simulink model "transmitSim"  (R2019a)
settings: Solver=VariableStepAuto  StartTime=0.0  StopTime=0.01  RelTol=1e-3
values from neighbouring files (symbols this model uses):
  data = 1:53    [cable.m]
libraries: commrandsrc3 x2, commdigbbndam3 x2, rfports1 x2, commchan3 x1, rftxlines1 x1
settings Model: Creator=PABLO  LastModifiedBy=PABLO

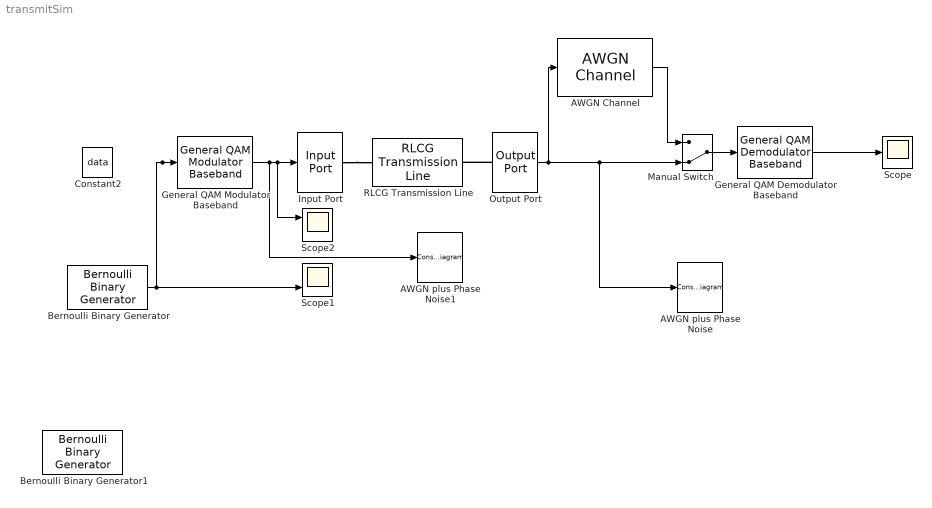
== system transmitSim ==
  AWGN Channel : commchan3/AWGN Channel  InputProcessing=Columns as channels (frame based)  seed=67  noiseMode="Signal to noise ratio  (Eb/No)"  EbNodB=10  EsNodB=10  SNRdB=10  bitsPerSym=1  Ps=1  Tsym=1  variance=1
      settings: SourceProductName=Communications Toolbox
  AWGN plus Phase Noise : ConstellationDiagram  Tag=ScatterPlot
  AWGN plus Phase Noise1 : ConstellationDiagram  Tag=ScatterPlot
  Bernoulli Binary Generator : commrandsrc3/Bernoulli Binary Generator  ProbabilityOfZero=0.5  SeedSource=Auto  Seed=0  SampleTime=1e-7  SamplesPerFrame=1  OutputDataType=double  SimulateUsing=Interpreted execution
      settings: SourceProductName=Communications Toolbox
  Bernoulli Binary Generator1 : commrandsrc3/Bernoulli Binary Generator  ProbabilityOfZero=0.5  SeedSource=Auto  Seed=0  SampleTime=1e-7  SamplesPerFrame=1  OutputDataType=boolean  SimulateUsing=Interpreted execution
      settings: SourceProductName=Communications Toolbox
  Constant2 : Constant  Value=data  VectorParams1D=off  OutDataTypeStr=double  SampleTime=1e-7
  General QAM Demodulator Baseband : commdigbbndam3/General QAM Demodulator Baseband  SigCon=[exp(2*pi*1i*[0:7]/8)]  OutType=Bit  DecType=Hard decision  VarSource=Dialog  Variance=1  outDtypeBit=boolean  outDtype=single  roundingMode=Floor  overflowMode=Wrap  OvFlMode=off  OvFlModeLastStrValue=off  sigConstWordLen=16  sigConstDataTypeStr=Inherit: Same word length as input  sigConstLastDataTypeStr=Inherit: Same word length as input  accum1WordLen=32  accum1FracLen=30  prodInWordLen=32  prodInFracLen=30  prodInDataTypeStr=Inherit: Same as accumulator 1  prodInLastDataTypeStr=Inherit: Same as accumulator 1  prodOutWordLen=32  prodOutFracLen=30  accum2WordLen=32  accum2FracLen=30  accum3WordLen=32  accum3FracLen=30  nsiWordLen=32  nsiFracLen=30  nsiDataTypeStr=Inherit: Same as accumulator 3  nsiLastDataTypeStr=Inherit: Same as accumulator 3  invn0WordLen=16  invn0FracLen=8  invn0DataTypeStr=Inherit: Same word length as input  invn0LastDataTypeStr=Inherit: Same word length as input  outputWordLen=32  outputFracLen=30
      settings: SourceProductName=Communications Toolbox  SourceProductBaseCode=CM
  General QAM Modulator Baseband : commdigbbndam3/General QAM Modulator Baseband  SigCon=[exp(2*pi*1i*[0:7]/8)]  outDtype=single  outWordLen=16  outUDDataType=sfix(16)  outFracLenMode=Best precision  outFracLen=15  outDataTypeStr=single  outLastDataTypeStr=single
      settings: SourceProductName=Communications Toolbox  SourceProductBaseCode=CM
  Input Port : rfports1/Input Port  Description=source block  TreatSimulinkInputSignalAs=Source voltage  MaxLength=128  FracBW=0  ModelDelay=0  Fc=2e9  Ts=1e-7  Zs=50  RFhasDSP=Elements as channels (sample based)  NoiseFlag=on  seed=67987  GoToTag=BAADJBMJMJMEIOSRFTJXVJV
      settings: SourceProductName=RF Blockset  SourceProductBaseCode=RB
  Manual Switch : ManualSwitch  CurrentSetting=0
  Output Port : rfports1/Output Port  Zl=50  Flag=1  num_Models=0  GoToTag=BAADJBMJMJMEIOSRFTJXVJV  PlotFreq=User-specified  SourceFreq=Derived from Input Port parameters  Freq=1e9:1e8:3e9  AllPlotType=X-Y plane  AppliedNetworkData=S11  AppliedComplexFormat=Magnitude (decibels)  AppliedNetworkData2=""  AppliedXParameter=Freq  AppliedXFormat=Hz  YOption=Linear  XOption=Linear  PlotZ0=50  DisplayData=off  NoBudgetPlot=Composite data  NetworkData=S11  SmithData=S11  PolarData=S11  ComplexFormat=Magnitude (decibels)  DBFormat=Magnitude (decibels)  DBMFormat=dBm  NoneFormat=None
      settings: SourceProductName=RF Blockset  SourceProductBaseCode=RB
  RLCG Transmission Line : rftxlines1/RLCG Transmission Line  LConnTagsString=__newl0  RConnTagsString=__newr0  R=0  L=0  C=0  G=0  ParamFreq=1e9  InterpMethod=Linear  LineLength=0.01  StubMode=Not a stub  Termination=Open  PlotFreq=User-specified  SourceFreq=User-specified  Freq=[1e9:1.0e6:3e9]  AllPlotType=X-Y plane  AppliedNetworkData=S21  AppliedComplexFormat=Angle (degrees)  AppliedNetworkData2=""  AppliedXParameter=Freq  AppliedXFormat=Hz  YOption=Linear  XOption=Linear  PlotZ0=50  DisplayData=off  PlotFreqNoSim=User-specified  NetworkData=S21  SmithData=S11  PolarData=S11  ComplexFormat=Angle  DBFormat=Magnitude (decibels)  NoneFormat=None
      settings: SourceProductName=RF Blockset  SourceProductBaseCode=RB
  Scope : Scope
  Scope1 : Scope  NumInputPorts=2
  Scope2 : Scope  NumInputPorts=2
  wires:
  Manual Switch/1 -> General QAM Demodulator Baseband/1
  Output Port/1 -> AWGN Channel/1, AWGN plus Phase Noise/1, Manual Switch/2
  AWGN Channel/1 -> Manual Switch/1
  General QAM Modulator Baseband/1 -> AWGN plus Phase Noise1/1, Scope2/1, Input Port/1
  General QAM Demodulator Baseband/1 -> Scope/1
  Bernoulli Binary Generator/1 -> Scope1/2, General QAM Modulator Baseband/1
  connections:
  Input Port/RConn1 -- RLCG Transmission Line/LConn1
  Output Port/LConn1 -- RLCG Transmission Line/RConn1
